simulink model "Q3"  (R2020b)
settings: Solver=VariableStepAuto  StartTime=0.0  StopTime=60  RelTol=1e-3
InitFcn:
  | H = 5;
  | Sb = 10000;
  | f0 = 50;
  | W0 = 100
  | DL = 1/200;
  | dPLoad = +1000
undefined symbols (not defined in the file): DL1, DL2, H1, H2, PT, R1, R2, Sb1, Sb2, Tturb1, Tturb2, W01, W02
Description:
  | Model of power system witthout control
  | Cretaed by Professor Francisco Gonzalez-Longatt
  | March 2021
settings Model: ModifiedHistory=Version 1: Created by Professor F. Gonzalez-Longatt 9 March 2021  Creator=fglon  LastModifiedBy=Dhanush Wagle

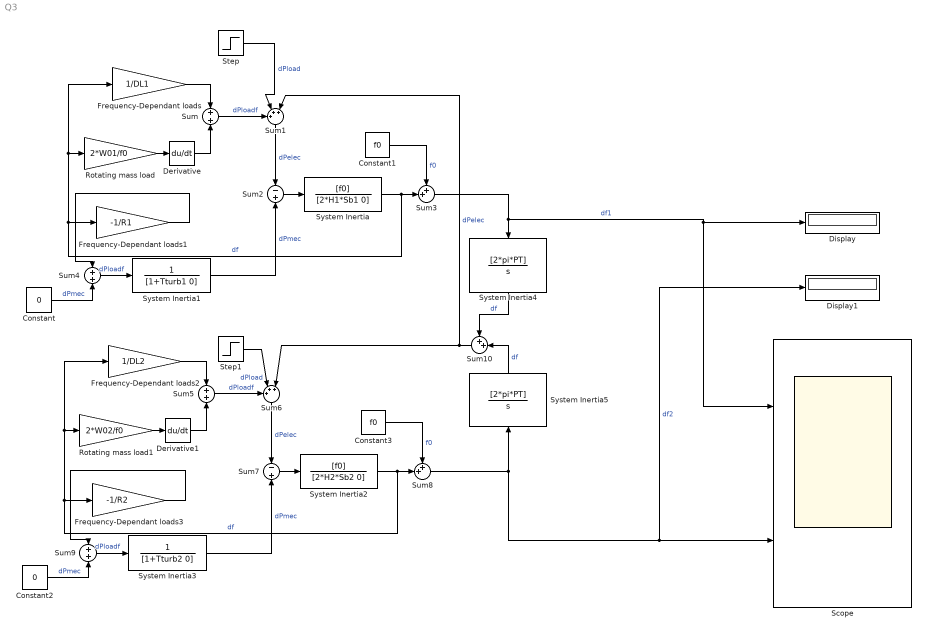
== system Q3 ==
  Constant : Constant  Value=0
  Constant1 : Constant  Value=f0
  Constant2 : Constant  Value=0
  Constant3 : Constant  Value=f0
  Derivative : Derivative
  Derivative1 : Derivative
  Display : Display
  Display1 : Display
  Frequency-Dependant loads : Gain  Gain=1/DL1
  Frequency-Dependant loads1 : Gain  Gain=-1/R1
  Frequency-Dependant loads2 : Gain  Gain=1/DL2
  Frequency-Dependant loads3 : Gain  Gain=-1/R2
  Rotating mass load : Gain  Gain=2*W01/f0
  Rotating mass load1 : Gain  Gain=2*W02/f0
  Scope : Scope  NumInputPorts=2
  Step : Step  After=100  SampleTime=0
  Step1 : Step  After=0  SampleTime=0
  Sum{,4..5,9} (4 alike) : Sum  Inputs=+|+
  Sum1 : Sum  Inputs=+++|
  Sum10 : Sum  Inputs=++|
  Sum2 : Sum  Inputs=-|+
  Sum3 : Sum  Inputs=++|
  Sum6 : Sum  Inputs=+++|
  Sum7 : Sum  Inputs=-|+
  Sum8 : Sum  Inputs=++|
  System Inertia : TransferFcn  Numerator=[f0]  Denominator=[2*H1*Sb1 0]
  System Inertia1 : TransferFcn  Denominator=[1+Tturb1 0]
  System Inertia2 : TransferFcn  Numerator=[f0]  Denominator=[2*H2*Sb2 0]
  System Inertia3 : TransferFcn  Denominator=[1+Tturb2 0]
  System Inertia4 : TransferFcn  Numerator=[2*pi*PT]  Denominator=[1 0]
  System Inertia5 : TransferFcn  Numerator=[2*pi*PT]  Denominator=[1 0]
  wires:
  Rotating mass load/1 -> Derivative/1
  Derivative/1 -> Sum/2
  Frequency-Dependant loads/1 -> Sum/1
  Sum/1 -> Sum1/1  "dPloadf"
  Step/1 -> Sum1/2  "dPload"
  Sum1/1 -> Sum2/1  "dPelec"
  Sum2/1 -> System Inertia/1
  System Inertia/1 -> Frequency-Dependant loads1/1, Frequency-Dependant loads/1, Rotating mass load/1, Sum3/2  "df"
  Constant1/1 -> Sum3/1  "f0"
  Sum4/1 -> System Inertia1/1  "dPloadf"
  Constant/1 -> Sum4/2  "dPmec"
  System Inertia1/1 -> Sum2/2  "dPmec"
  Frequency-Dependant loads1/1 -> Sum4/1
  Constant2/1 -> Sum9/2  "dPmec"
  Rotating mass load1/1 -> Derivative1/1
  Sum9/1 -> System Inertia3/1  "dPloadf"
  System Inertia3/1 -> Sum7/2  "dPmec"
  Sum7/1 -> System Inertia2/1
  Sum5/1 -> Sum6/1  "dPloadf"
  System Inertia2/1 -> Frequency-Dependant loads3/1, Frequency-Dependant loads2/1, Rotating mass load1/1, Sum8/2  "df"
  Sum6/1 -> Sum7/1  "dPelec"
  Step1/1 -> Sum6/2  "dPload"
  Frequency-Dependant loads2/1 -> Sum5/1
  Derivative1/1 -> Sum5/2
  Constant3/1 -> Sum8/1  "f0"
  Frequency-Dependant loads3/1 -> Sum9/1
  Sum3/1 -> System Inertia4/1, Scope/1, Display/1  "df1"
  Sum8/1 -> System Inertia5/1, Display1/1, Scope/2  "df2"
  System Inertia5/1 -> Sum10/2  "df"
  System Inertia4/1 -> Sum10/1  "df"
  Sum10/1 -> Sum6/3, Sum1/3  "dPelec"
